simulink model "HarrierLateral"  (R2020a)
settings: Solver=VariableStepAuto  StartTime=0.0  StopTime=50  RelTol=1e-3
values from neighbouring files (symbols this model uses):
  A = [0, 0, 1, 0 ... (first row only)    [HarrierLateralController.m]    (also in HarrierVerticalController.m)
  B = [0 ... (first row only)    [HarrierLateralController.m]    (also in HarrierVerticalController.m)
  C = [1, 0, 0, 0]    [HarrierLateralController.m]    (also in HarrierVerticalController.m = [1, 0, 0, 0, 0, 0)
  K = [0.8,1,1,1].*K    [HarrierLateralController.m]    (also in HarrierVerticalController.m = place(A,B,roots_scaled))
  kr = 1/(C*inv(A-B*K)*B)    [HarrierLateralController.m]    (also in HarrierVerticalController.m = kr(1,1))
  L = K'    [HarrierLateralController.m]    (also in HarrierVerticalController.m = place(A',C',roots_scaled)')
  m = 22471    [HarrierLateralController.m]    (also in HarrierVerticalController.m)
  r = 0    [HarrierLateralController.m]    (also in HarrierVerticalController.m = [5*WS, 0, 0, 0])
settings Model: Creator=oscar  LastModifiedBy=Finn
settings DebuggingCC: SFMachineParentedDataDiag=error

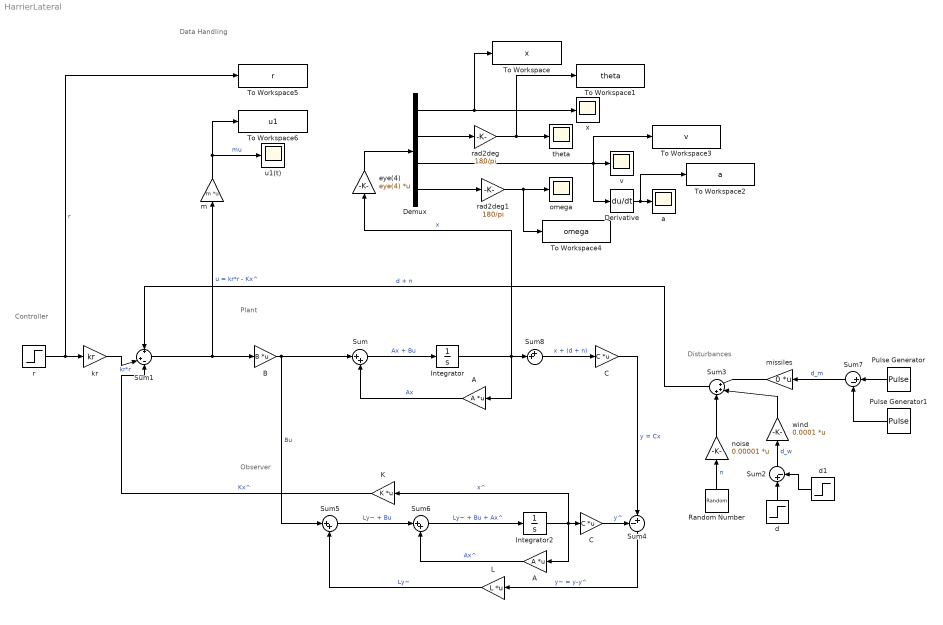
== system HarrierLateral ==
  note: Controller
  note: Plant
  note: Data Handling
  note: Disturbances
  note: Observer
  " L" : Gain  Gain=L  Multiplication=Matrix(K*u)
  A : Gain  Gain=A  Multiplication=Matrix(K*u)
  "A " : Gain  Gain=A  Multiplication=Matrix(K*u)
  "B " : Gain  Gain=B  Multiplication=Matrix(K*u)
  C : Gain  Gain=C  Multiplication=Matrix(K*u)
  "C " : Gain  Gain=C  Multiplication=Matrix(K*u)
  Demux : Demux
  Derivative : Derivative
  Integrator : Integrator
  Integrator2 : Integrator
  "K " : Gain  Gain=K  Multiplication=Matrix(K*u)
  Pulse Generator : DiscretePulseGenerator  PulseType=Time based  Period=10  PulseWidth=2
  Pulse Generator1 : DiscretePulseGenerator  PulseType=Time based  Period=10  PulseWidth=2  PhaseDelay=40
  Random Number : RandomNumber  Variance=0.8  Seed=420  SampleTime=0.05
  Sum : Sum  Inputs=|++
  Sum1 : Sum  Inputs=+|+-
  Sum2 : Sum  Inputs=|+-
  Sum3 : Sum  Inputs=|+++
  Sum4 : Sum  Inputs=-+|
  Sum5 : Sum  Inputs=|++
  Sum6 : Sum  Inputs=|++
  Sum7 : Sum  Inputs=|+-
  Sum8 : Sum  Inputs=++|
  To Workspace : ToWorkspace  VariableName=x  SampleTime=-1
  To Workspace1 : ToWorkspace  VariableName=theta  SampleTime=-1
  To Workspace2 : ToWorkspace  VariableName=a  SampleTime=-1
  To Workspace3 : ToWorkspace  VariableName=v  SampleTime=-1
  To Workspace4 : ToWorkspace  VariableName=omega  SampleTime=-1
  To Workspace5 : ToWorkspace  VariableName=r  SampleTime=-1
  To Workspace6 : ToWorkspace  VariableName=u1  SampleTime=-1
  a : Scope
  d : Step  Time=5  SampleTime=0
  d1 : Step  Time=30  SampleTime=0
  eye(4) : Gain  Gain=eye(4)  Multiplication=Matrix(K*u)
  kr : Gain  Gain=kr
  m : Gain  Gain=m  Multiplication=Matrix(K*u)
  missiles : Gain  Gain=0  Multiplication=Matrix(K*u)
  noise : Gain  Gain=0.00001  Multiplication=Matrix(K*u)
  omega : Scope
  r : Step  After=r  SampleTime=0
  rad2deg : Gain  Gain=180/pi
  rad2deg1 : Gain  Gain=180/pi
  theta : Scope
  u1(t) : Scope
  v : Scope
  wind : Gain  Gain=0.0001  Multiplication=Matrix(K*u)
  x : Scope
  wires:
  r/1 -> kr/1, To Workspace5/1  "r"
  Sum1/1 -> m/1, "B "/1  "u = kr*r - Kx^"
  "B "/1 -> Sum/1, Sum5/1  "Bu"
  A/1 -> Sum/2  "Ax"
  kr/1 -> Sum1/2  "kr*r"
  m/1 -> To Workspace6/1, u1(t)/1  "mu"
  Integrator/1 -> Sum8/2, eye(4)/1, A/1  "x"
  "C "/1 -> Sum4/2  "y = Cx"
  Sum4/1 -> " L"/1  "y~ = y-y^"
  Sum5/1 -> Sum6/1  "Ly~ + Bu"
  "A "/1 -> Sum6/2  "Ax^"
  Sum6/1 -> Integrator2/1  "Ly~ + Bu + Ax^"
  Integrator2/1 -> "A "/1, "K "/1, C/1  "x^"
  "K "/1 -> Sum1/3  "Kx^"
  C/1 -> Sum4/1  "y^"
  rad2deg/1 -> To Workspace1/1, theta/1
  Derivative/1 -> To Workspace2/1, a/1
  rad2deg1/1 -> To Workspace4/1, omega/1
  Demux/4 -> rad2deg1/1
  Demux/2 -> rad2deg/1
  Demux/1 -> x/1, To Workspace/1
  Demux/3 -> To Workspace3/1, Derivative/1, v/1
  eye(4)/1 -> Demux/1
  Random Number/1 -> noise/1  "n"
  missiles/1 -> Sum3/1
  Sum2/1 -> wind/1  "d_w"
  d/1 -> Sum2/1
  d1/1 -> Sum2/2
  wind/1 -> Sum3/2
  Pulse Generator1/1 -> Sum7/2
  Pulse Generator/1 -> Sum7/1
  Sum7/1 -> missiles/1  "d_m"
  " L"/1 -> Sum5/2  "Ly~"
  Sum/1 -> Integrator/1  "Ax + Bu"
  noise/1 -> Sum3/3
  Sum8/1 -> "C "/1  "x + (d + n)"
  Sum3/1 -> Sum1/1  "d + n"
